simulink model "soal5_C"  (R2021b)
settings: Solver=VariableStepAuto  StartTime=0.0  StopTime=10.0  RelTol=1e-3
settings Model: Creator=Homa Rayaneh  LastModifiedBy=Homa Rayaneh

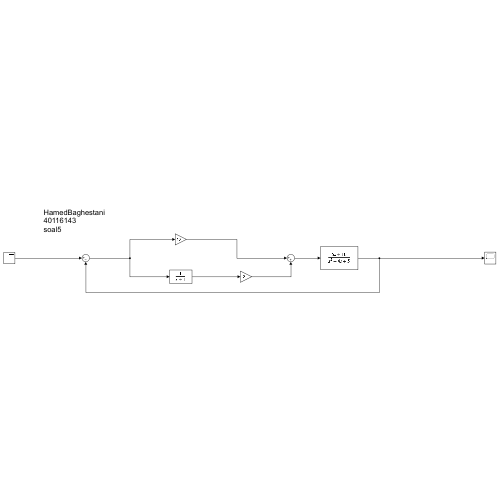
[thumbnail: Simulink's stored preview of the top-level diagram]
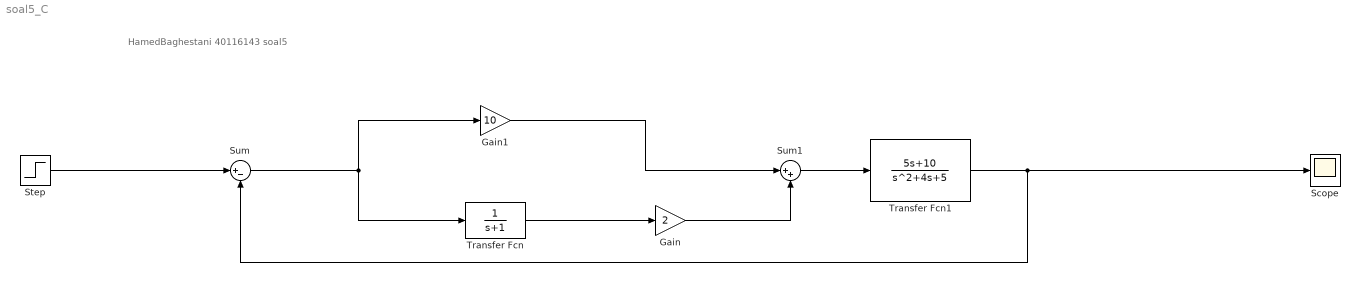
== system soal5_C ==
  note: HamedBaghestani
      | 40116143
      | soal5
  Gain : Gain  Gain=2
  Gain1 : Gain  Gain=10
  Scope : Scope
  Step : Step  Time=0  SampleTime=0
  Sum : Sum  Inputs=|+-
  Sum1 : Sum  Inputs=|++
  Transfer Fcn : TransferFcn  Denominator=[1 1]
  Transfer Fcn1 : TransferFcn  Numerator=[5 10]  Denominator=[1 4 5]
  wires:
  Step/1 -> Sum/1
  Sum/1 -> Gain1/1, Transfer Fcn/1
  Transfer Fcn/1 -> Gain/1
  Transfer Fcn1/1 -> Sum/2, Scope/1
  Sum1/1 -> Transfer Fcn1/1
  Gain/1 -> Sum1/2
  Gain1/1 -> Sum1/1
